simulink model "GPI1"  (Simulink 7.0)
settings: Solver=ode45  StartTime=0.0  StopTime=1000.0  RelTol=1e-3
values from neighbouring files (symbols this model uses):
  A_gpegpi = 1    [data_GPE.m]    (also in data_GPI.m)
  A_gpi = 2    [data_GPI.m]
  A_stngpi = 1    [data_GPI.m]    (also in data_STN.m)
  B_gpegpi = .1    (= 0.1)    [data_GPE.m]    (also in data_GPI.m)
  B_gpi = .08    (= 0.08)    [data_GPI.m]
  B_stngpi = .05    (= 0.05)    [data_GPI.m]    (also in data_STN.m)
  c_gpi = 1    [data_GPI.m]
  cagi0 = i_v_16(289:304)    [launch_sysGPI_mod.m]
  egpegpi = -100    [data_synapses.m]
  ek_gpi = -80.0    (= -80)    [data_GPI.m]
  el_gpi = -55.0    (= -55)    [data_GPI.m]
  epsil_gpi = 1*10^-4    (= 0.0001)    [data_GPI.m]
  estngpi = 0    [data_synapses.m]
  gahp_gpi = 30.0    (= 30)    [data_GPI.m]
  gca_gpi = 0.15    [data_GPI.m]
  ggpegpi = ggpegpi_vec(i)    [CN_launch_CN_analyze_TAL2.m]    (also in data_synapses.m = 1; launch_sysGPI_mod.m = 0.3)
  gk_gpi = 30.0    (= 30)    [data_GPI.m]
  gl_gpi = .1    (= 0.1)    [data_GPI.m]
  gna_gpi = 120    [data_GPI.m]
  gstngpi = .3    (= 0.3)    [data_synapses.m]
  gt_gpi = .5    (= 0.5)    [data_GPI.m]
  hgi0 = i_v_16(241:256)    [launch_sysGPI_mod.m]
  k1_gpi = 30.0    (= 30)    [data_GPI.m]
  kca_gpi = 15    [data_GPI.m]
  ngi0 = i_v_16(257:272)    [launch_sysGPI_mod.m]
  phih_gpi = 0.05    [data_GPI.m]
  phin_gpi = 0.1    [data_GPI.m]
  phir_gpi = 1    [data_GPI.m]
  rgi0 = i_v_16(273:288)    [launch_sysGPI_mod.m]
  sgi0 = i_v_16(305:320)    [launch_sysGPI_mod.m]
  sig0 = i_v_16(209:224)    [launch_sysGPI_mod.m]
  sigmaa_gpi = 2    [data_GPI.m]
  sigmagh_gpe = 2.0    (= 2)    [data_GPE.m]
  sigmagh_gpi = 2.0    (= 2)    [data_GPI.m]
  sigmagh_stn = 8.0    (= 8)    [data_STN.m]
  sigmah_gpi = -12    [data_GPI.m]
  sigmam_gpi = 10.0    (= 10)    [data_GPI.m]
  sigman_gpi = 14.0    (= 14)    [data_GPI.m]
  sigmar_gpi = -2.0    (= -2)    [data_GPI.m]
  sigmas_gpi = 2    [data_GPI.m]
  sigmatauh_gpi = -12    [data_GPI.m]
  sigmataun_gpi = -12.0    (= -12)    [data_GPI.m]
  sis0 = i_v_16(97:112)    [launch_sysGPI_mod.m]
  tauh0_gpi = .05    (= 0.05)    [data_GPI.m]
  tauh1_gpi = .27    (= 0.27)    [data_GPI.m]
  taun0_gpi = .05    (= 0.05)    [data_GPI.m]
  taun1_gpi = .27    (= 0.27)    [data_GPI.m]
  taur_gpi = 30.0    (= 30)    [data_GPI.m]
  theta_gpe = 20    [data_GPE.m]    (also in data_GPI.m)
  theta_gpi = 20    [data_GPI.m]
  theta_stn = 30    [data_GPI.m]    (also in data_STN.m)
  thetaa_gpi = -57.0    (= -57)    [data_GPI.m]
  thetagh_gpe = -57.0    (= -57)    [data_GPE.m]
  thetagh_gpi = -57.0    (= -57)    [data_GPI.m]
  thetagh_stn = -39.0    (= -39)    [data_STN.m]
  thetah_gpi = -58.0    (= -58)    [data_GPI.m]
  thetam_gpi = -37.0    (= -37)    [data_GPI.m]
  thetan_gpi = -50.0    (= -50)    [data_GPI.m]
  thetar_gpi = -70.0    (= -70)    [data_GPI.m]
  thetas_gpi = -35.0    (= -35)    [data_GPI.m]
  thetatauh_gpi = -40.0    (= -40)    [data_GPI.m]
  thetataun_gpi = -40.0    (= -40)    [data_GPI.m]
  vgi0 = i_v_16(225:240)    [launch_sysGPI_mod.m]
(part 6 of 6)

== system GPI1/gpicomp3/gpi_cell/ina/ina_gpi ==
  In1 : Inport  OutDataType=sfix(16)  OutScaling=2^0
  In2 : Inport  Port=2  OutDataType=sfix(16)  OutScaling=2^0
  In3 : Inport  Port=3  OutDataType=sfix(16)  OutScaling=2^0
  Fcn1 : Fcn  Expr=u^3*gna_gpi
  Fcn2 : Fcn  Expr=u-ena_gpi
  Product : Product  Inputs=3  OutDataType=sfix(16)  OutScaling=2^0  SaturateOnIntegerOverflow=on  InputSameDT=on
  Out1 : Outport  OutDataType=sfix(16)  OutScaling=2^0
  wires:
  Fcn1/1 -> Product/2
  Fcn2/1 -> Product/1
  In1/1 -> Fcn2/1
  Product/1 -> Out1/1
  In3/1 -> Product/3
  In2/1 -> Fcn1/1

== system GPI1/gpicomp3/gpi_cell/it/it_gpi ==
  In1 : Inport  OutDataType=sfix(16)  OutScaling=2^0
  In2 : Inport  Port=2  OutDataType=sfix(16)  OutScaling=2^0
  In3 : Inport  Port=3  OutDataType=sfix(16)  OutScaling=2^0
  Fcn1 : Fcn  Expr=u^2*gt_gpi
  Fcn2 : Fcn  Expr=u-eca_gpi
  Fcn3 : Fcn  Expr=u^3
  Product : Product  Inputs=3  OutDataType=sfix(16)  OutScaling=2^0  SaturateOnIntegerOverflow=on  InputSameDT=on
  Out1 : Outport  OutDataType=sfix(16)  OutScaling=2^0
  wires:
  Fcn1/1 -> Product/2
  Fcn2/1 -> Product/1
  In1/1 -> Fcn2/1
  Product/1 -> Out1/1
  In2/1 -> Fcn1/1
  In3/1 -> Fcn3/1
  Fcn3/1 -> Product/3

== system GPI1/gpicomp3/gpi_cell/it/r_gpi ==
  In1 : Inport  OutDataType=sfix(16)  OutScaling=2^0
  In2 : Inport  Port=2  OutDataType=sfix(16)  OutScaling=2^0
  1/tau_r : Fcn  Expr=1/taur_gpi
  Gain : Gain  Gain=phir_gpi  ParameterDataType=sfix(16)  ParameterScaling=2^0  OutDataType=sfix(16)  OutScaling=2^0  SaturateOnIntegerOverflow=on
  Integrator1 : Integrator  InitialConditionSource=external
  Product : Product  OutDataType=sfix(16)  OutScaling=2^0  SaturateOnIntegerOverflow=on  InputSameDT=on
  Sum1 : Sum  Inputs=|+-  OutDataType=sfix(16)  OutScaling=2^0  SaturateOnIntegerOverflow=on  InputSameDT=on
  rinf : Fcn  Expr=1/(1 + exp(-(u-thetar_gpi)/sigmar_gpi))
  Out1 : Outport  OutDataType=sfix(16)  OutScaling=2^0
  wires:
  In1/1 -> 1/tau_r/1, rinf/1
  1/tau_r/1 -> Product/1
  Integrator1/1 -> Sum1/2, Out1/1
  rinf/1 -> Sum1/1
  Sum1/1 -> Product/2
  Product/1 -> Gain/1
  Gain/1 -> Integrator1/1
  In2/1 -> Integrator1/2

== system GPI1/gpicomp4/gpi_cell/iahp/Subsystem ==
  In1 : Inport  OutDataType=sfix(16)  OutScaling=2^0
  In2 : Inport  Port=2  OutDataType=sfix(16)  OutScaling=2^0
  In3 : Inport  Port=3  OutDataType=sfix(16)  OutScaling=2^0
  Gain1 : Gain  Gain=epsil_gpi  ParameterDataType=sfix(16)  ParameterScaling=2^0  OutDataType=sfix(16)  OutScaling=2^0  SaturateOnIntegerOverflow=on
  Gain2 : Gain  Orientation=left  Gain=kca_gpi  ParameterDataType=sfix(16)  ParameterScaling=2^0  OutDataType=sfix(16)  OutScaling=2^0  SaturateOnIntegerOverflow=on
  Integrator1 : Integrator  InitialConditionSource=external  InitialCondition=0.03
  Sum1 : Sum  Inputs=---  OutDataType=sfix(16)  OutScaling=2^0  SaturateOnIntegerOverflow=on  InputSameDT=on
  Out1 : Outport  OutDataType=sfix(16)  OutScaling=2^0
  wires:
  Sum1/1 -> Gain1/1
  Gain1/1 -> Integrator1/1
  Gain2/1 -> Sum1/3
  Integrator1/1 -> Out1/1, Gain2/1
  In1/1 -> Sum1/1
  In2/1 -> Sum1/2
  In3/1 -> Integrator1/2

== system GPI1/gpicomp4/gpi_cell/ica/ica_gpe ==
  In1 : Inport  OutDataType=sfix(16)  OutScaling=2^0
  In2 : Inport  Port=2  OutDataType=sfix(16)  OutScaling=2^0
  Fcn1 : Fcn  Expr=u^2*gca_gpi
  Fcn2 : Fcn  Expr=u-eca_gpi
  Product : Product  OutDataType=sfix(16)  OutScaling=2^0  SaturateOnIntegerOverflow=on  InputSameDT=on
  Out1 : Outport  OutDataType=sfix(16)  OutScaling=2^0
  wires:
  Fcn1/1 -> Product/2
  Fcn2/1 -> Product/1
  In1/1 -> Fcn2/1
  Product/1 -> Out1/1
  In2/1 -> Fcn1/1

== system GPI1/gpicomp4/gpi_cell/ik/ik_gpi ==
  In1 : Inport  OutDataType=sfix(16)  OutScaling=2^0
  In2 : Inport  Port=2  OutDataType=sfix(16)  OutScaling=2^0
  Fcn1 : Fcn  Expr=u^4*gk_gpi
  Fcn2 : Fcn  Expr=u-ek_gpi
  Product : Product  OutDataType=sfix(16)  OutScaling=2^0  SaturateOnIntegerOverflow=on  InputSameDT=on
  Out1 : Outport  OutDataType=sfix(16)  OutScaling=2^0
  wires:
  Fcn1/1 -> Product/2
  Fcn2/1 -> Product/1
  In1/1 -> Fcn2/1
  Product/1 -> Out1/1
  In2/1 -> Fcn1/1

== system GPI1/gpicomp4/gpi_cell/ik/n_gpi ==
  In1 : Inport  OutDataType=sfix(16)  OutScaling=2^0
  In2 : Inport  Port=2  OutDataType=sfix(16)  OutScaling=2^0
  1/tau_n : Fcn  Expr=1/(taun0_gpi+ taun1_gpi/(1+exp(-(u-thetataun_gpi)/sigmataun_gpi)))
  Gain : Gain  Gain=phin_gpi  ParameterDataType=sfix(16)  ParameterScaling=2^0  OutDataType=sfix(16)  OutScaling=2^0  SaturateOnIntegerOverflow=on
  Integrator1 : Integrator  InitialConditionSource=external
  Product : Product  OutDataType=sfix(16)  OutScaling=2^0  SaturateOnIntegerOverflow=on  InputSameDT=on
  Sum1 : Sum  Inputs=|+-  OutDataType=sfix(16)  OutScaling=2^0  SaturateOnIntegerOverflow=on  InputSameDT=on
  ninf : Fcn  Expr=1/(1 + exp(-(u-thetan_gpi)/sigman_gpi))
  Out1 : Outport  OutDataType=sfix(16)  OutScaling=2^0
  wires:
  In1/1 -> 1/tau_n/1, ninf/1
  1/tau_n/1 -> Product/1
  Integrator1/1 -> Sum1/2, Out1/1
  ninf/1 -> Sum1/1
  Sum1/1 -> Product/2
  Product/1 -> Gain/1
  Gain/1 -> Integrator1/1
  In2/1 -> Integrator1/2

== system GPI1/gpicomp4/gpi_cell/ina/h_gpi ==
  In1 : Inport  OutDataType=sfix(16)  OutScaling=2^0
  In2 : Inport  Port=2  OutDataType=sfix(16)  OutScaling=2^0
  1/tau_h : Fcn  Expr=1/(tauh0_gpi + tauh1_gpi/(1+exp(-(u-thetatauh_gpi)/sigmatauh_gpi)))
  Gain : Gain  Gain=phih_gpi  ParameterDataType=sfix(16)  ParameterScaling=2^0  OutDataType=sfix(16)  OutScaling=2^0  SaturateOnIntegerOverflow=on
  Integrator1 : Integrator  InitialConditionSource=external
  Product : Product  OutDataType=sfix(16)  OutScaling=2^0  SaturateOnIntegerOverflow=on  InputSameDT=on
  Sum1 : Sum  Inputs=|+-  OutDataType=sfix(16)  OutScaling=2^0  SaturateOnIntegerOverflow=on  InputSameDT=on
  hinf : Fcn  Expr=1/(1 + exp(-(u-thetah_gpi)/sigmah_gpi))
  Out1 : Outport  OutDataType=sfix(16)  OutScaling=2^0
  wires:
  In1/1 -> 1/tau_h/1, hinf/1
  1/tau_h/1 -> Product/1
  Integrator1/1 -> Sum1/2, Out1/1
  hinf/1 -> Sum1/1
  Sum1/1 -> Product/2
  Product/1 -> Gain/1
  Gain/1 -> Integrator1/1
  In2/1 -> Integrator1/2

== system GPI1/gpicomp4/gpi_cell/ina/ina_gpi ==
  In1 : Inport  OutDataType=sfix(16)  OutScaling=2^0
  In2 : Inport  Port=2  OutDataType=sfix(16)  OutScaling=2^0
  In3 : Inport  Port=3  OutDataType=sfix(16)  OutScaling=2^0
  Fcn1 : Fcn  Expr=u^3*gna_gpi
  Fcn2 : Fcn  Expr=u-ena_gpi
  Product : Product  Inputs=3  OutDataType=sfix(16)  OutScaling=2^0  SaturateOnIntegerOverflow=on  InputSameDT=on
  Out1 : Outport  OutDataType=sfix(16)  OutScaling=2^0
  wires:
  Fcn1/1 -> Product/2
  Fcn2/1 -> Product/1
  In1/1 -> Fcn2/1
  Product/1 -> Out1/1
  In3/1 -> Product/3
  In2/1 -> Fcn1/1

== system GPI1/gpicomp4/gpi_cell/it/it_gpi ==
  In1 : Inport  OutDataType=sfix(16)  OutScaling=2^0
  In2 : Inport  Port=2  OutDataType=sfix(16)  OutScaling=2^0
  In3 : Inport  Port=3  OutDataType=sfix(16)  OutScaling=2^0
  Fcn1 : Fcn  Expr=u^2*gt_gpi
  Fcn2 : Fcn  Expr=u-eca_gpi
  Fcn3 : Fcn  Expr=u^3
  Product : Product  Inputs=3  OutDataType=sfix(16)  OutScaling=2^0  SaturateOnIntegerOverflow=on  InputSameDT=on
  Out1 : Outport  OutDataType=sfix(16)  OutScaling=2^0
  wires:
  Fcn1/1 -> Product/2
  Fcn2/1 -> Product/1
  In1/1 -> Fcn2/1
  Product/1 -> Out1/1
  In2/1 -> Fcn1/1
  In3/1 -> Fcn3/1
  Fcn3/1 -> Product/3

== system GPI1/gpicomp4/gpi_cell/it/r_gpi ==
  In1 : Inport  OutDataType=sfix(16)  OutScaling=2^0
  In2 : Inport  Port=2  OutDataType=sfix(16)  OutScaling=2^0
  1/tau_r : Fcn  Expr=1/taur_gpi
  Gain : Gain  Gain=phir_gpi  ParameterDataType=sfix(16)  ParameterScaling=2^0  OutDataType=sfix(16)  OutScaling=2^0  SaturateOnIntegerOverflow=on
  Integrator1 : Integrator  InitialConditionSource=external
  Product : Product  OutDataType=sfix(16)  OutScaling=2^0  SaturateOnIntegerOverflow=on  InputSameDT=on
  Sum1 : Sum  Inputs=|+-  OutDataType=sfix(16)  OutScaling=2^0  SaturateOnIntegerOverflow=on  InputSameDT=on
  rinf : Fcn  Expr=1/(1 + exp(-(u-thetar_gpi)/sigmar_gpi))
  Out1 : Outport  OutDataType=sfix(16)  OutScaling=2^0
  wires:
  In1/1 -> 1/tau_r/1, rinf/1
  1/tau_r/1 -> Product/1
  Integrator1/1 -> Sum1/2, Out1/1
  rinf/1 -> Sum1/1
  Sum1/1 -> Product/2
  Product/1 -> Gain/1
  Gain/1 -> Integrator1/1
  In2/1 -> Integrator1/2

== system GPI1/gpicomp5/gpi_cell/iahp/Subsystem ==
  In1 : Inport  OutDataType=sfix(16)  OutScaling=2^0
  In2 : Inport  Port=2  OutDataType=sfix(16)  OutScaling=2^0
  In3 : Inport  Port=3  OutDataType=sfix(16)  OutScaling=2^0
  Gain1 : Gain  Gain=epsil_gpi  ParameterDataType=sfix(16)  ParameterScaling=2^0  OutDataType=sfix(16)  OutScaling=2^0  SaturateOnIntegerOverflow=on
  Gain2 : Gain  Orientation=left  Gain=kca_gpi  ParameterDataType=sfix(16)  ParameterScaling=2^0  OutDataType=sfix(16)  OutScaling=2^0  SaturateOnIntegerOverflow=on
  Integrator1 : Integrator  InitialConditionSource=external  InitialCondition=0.03
  Sum1 : Sum  Inputs=---  OutDataType=sfix(16)  OutScaling=2^0  SaturateOnIntegerOverflow=on  InputSameDT=on
  Out1 : Outport  OutDataType=sfix(16)  OutScaling=2^0
  wires:
  Sum1/1 -> Gain1/1
  Gain1/1 -> Integrator1/1
  Gain2/1 -> Sum1/3
  Integrator1/1 -> Out1/1, Gain2/1
  In1/1 -> Sum1/1
  In2/1 -> Sum1/2
  In3/1 -> Integrator1/2

== system GPI1/gpicomp5/gpi_cell/ica/ica_gpe ==
  In1 : Inport  OutDataType=sfix(16)  OutScaling=2^0
  In2 : Inport  Port=2  OutDataType=sfix(16)  OutScaling=2^0
  Fcn1 : Fcn  Expr=u^2*gca_gpi
  Fcn2 : Fcn  Expr=u-eca_gpi
  Product : Product  OutDataType=sfix(16)  OutScaling=2^0  SaturateOnIntegerOverflow=on  InputSameDT=on
  Out1 : Outport  OutDataType=sfix(16)  OutScaling=2^0
  wires:
  Fcn1/1 -> Product/2
  Fcn2/1 -> Product/1
  In1/1 -> Fcn2/1
  Product/1 -> Out1/1
  In2/1 -> Fcn1/1

== system GPI1/gpicomp5/gpi_cell/ik/ik_gpi ==
  In1 : Inport  OutDataType=sfix(16)  OutScaling=2^0
  In2 : Inport  Port=2  OutDataType=sfix(16)  OutScaling=2^0
  Fcn1 : Fcn  Expr=u^4*gk_gpi
  Fcn2 : Fcn  Expr=u-ek_gpi
  Product : Product  OutDataType=sfix(16)  OutScaling=2^0  SaturateOnIntegerOverflow=on  InputSameDT=on
  Out1 : Outport  OutDataType=sfix(16)  OutScaling=2^0
  wires:
  Fcn1/1 -> Product/2
  Fcn2/1 -> Product/1
  In1/1 -> Fcn2/1
  Product/1 -> Out1/1
  In2/1 -> Fcn1/1

== system GPI1/gpicomp5/gpi_cell/ik/n_gpi ==
  In1 : Inport  OutDataType=sfix(16)  OutScaling=2^0
  In2 : Inport  Port=2  OutDataType=sfix(16)  OutScaling=2^0
  1/tau_n : Fcn  Expr=1/(taun0_gpi+ taun1_gpi/(1+exp(-(u-thetataun_gpi)/sigmataun_gpi)))
  Gain : Gain  Gain=phin_gpi  ParameterDataType=sfix(16)  ParameterScaling=2^0  OutDataType=sfix(16)  OutScaling=2^0  SaturateOnIntegerOverflow=on
  Integrator1 : Integrator  InitialConditionSource=external
  Product : Product  OutDataType=sfix(16)  OutScaling=2^0  SaturateOnIntegerOverflow=on  InputSameDT=on
  Sum1 : Sum  Inputs=|+-  OutDataType=sfix(16)  OutScaling=2^0  SaturateOnIntegerOverflow=on  InputSameDT=on
  ninf : Fcn  Expr=1/(1 + exp(-(u-thetan_gpi)/sigman_gpi))
  Out1 : Outport  OutDataType=sfix(16)  OutScaling=2^0
  wires:
  In1/1 -> 1/tau_n/1, ninf/1
  1/tau_n/1 -> Product/1
  Integrator1/1 -> Sum1/2, Out1/1
  ninf/1 -> Sum1/1
  Sum1/1 -> Product/2
  Product/1 -> Gain/1
  Gain/1 -> Integrator1/1
  In2/1 -> Integrator1/2

== system GPI1/gpicomp5/gpi_cell/ina/h_gpi ==
  In1 : Inport  OutDataType=sfix(16)  OutScaling=2^0
  In2 : Inport  Port=2  OutDataType=sfix(16)  OutScaling=2^0
  1/tau_h : Fcn  Expr=1/(tauh0_gpi + tauh1_gpi/(1+exp(-(u-thetatauh_gpi)/sigmatauh_gpi)))
  Gain : Gain  Gain=phih_gpi  ParameterDataType=sfix(16)  ParameterScaling=2^0  OutDataType=sfix(16)  OutScaling=2^0  SaturateOnIntegerOverflow=on
  Integrator1 : Integrator  InitialConditionSource=external
  Product : Product  OutDataType=sfix(16)  OutScaling=2^0  SaturateOnIntegerOverflow=on  InputSameDT=on
  Sum1 : Sum  Inputs=|+-  OutDataType=sfix(16)  OutScaling=2^0  SaturateOnIntegerOverflow=on  InputSameDT=on
  hinf : Fcn  Expr=1/(1 + exp(-(u-thetah_gpi)/sigmah_gpi))
  Out1 : Outport  OutDataType=sfix(16)  OutScaling=2^0
  wires:
  In1/1 -> 1/tau_h/1, hinf/1
  1/tau_h/1 -> Product/1
  Integrator1/1 -> Sum1/2, Out1/1
  hinf/1 -> Sum1/1
  Sum1/1 -> Product/2
  Product/1 -> Gain/1
  Gain/1 -> Integrator1/1
  In2/1 -> Integrator1/2

== system GPI1/gpicomp5/gpi_cell/ina/ina_gpi ==
  In1 : Inport  OutDataType=sfix(16)  OutScaling=2^0
  In2 : Inport  Port=2  OutDataType=sfix(16)  OutScaling=2^0
  In3 : Inport  Port=3  OutDataType=sfix(16)  OutScaling=2^0
  Fcn1 : Fcn  Expr=u^3*gna_gpi
  Fcn2 : Fcn  Expr=u-ena_gpi
  Product : Product  Inputs=3  OutDataType=sfix(16)  OutScaling=2^0  SaturateOnIntegerOverflow=on  InputSameDT=on
  Out1 : Outport  OutDataType=sfix(16)  OutScaling=2^0
  wires:
  Fcn1/1 -> Product/2
  Fcn2/1 -> Product/1
  In1/1 -> Fcn2/1
  Product/1 -> Out1/1
  In3/1 -> Product/3
  In2/1 -> Fcn1/1

== system GPI1/gpicomp5/gpi_cell/it/it_gpi ==
  In1 : Inport  OutDataType=sfix(16)  OutScaling=2^0
  In2 : Inport  Port=2  OutDataType=sfix(16)  OutScaling=2^0
  In3 : Inport  Port=3  OutDataType=sfix(16)  OutScaling=2^0
  Fcn1 : Fcn  Expr=u^2*gt_gpi
  Fcn2 : Fcn  Expr=u-eca_gpi
  Fcn3 : Fcn  Expr=u^3
  Product : Product  Inputs=3  OutDataType=sfix(16)  OutScaling=2^0  SaturateOnIntegerOverflow=on  InputSameDT=on
  Out1 : Outport  OutDataType=sfix(16)  OutScaling=2^0
  wires:
  Fcn1/1 -> Product/2
  Fcn2/1 -> Product/1
  In1/1 -> Fcn2/1
  Product/1 -> Out1/1
  In2/1 -> Fcn1/1
  In3/1 -> Fcn3/1
  Fcn3/1 -> Product/3

== system GPI1/gpicomp5/gpi_cell/it/r_gpi ==
  In1 : Inport  OutDataType=sfix(16)  OutScaling=2^0
  In2 : Inport  Port=2  OutDataType=sfix(16)  OutScaling=2^0
  1/tau_r : Fcn  Expr=1/taur_gpi
  Gain : Gain  Gain=phir_gpi  ParameterDataType=sfix(16)  ParameterScaling=2^0  OutDataType=sfix(16)  OutScaling=2^0  SaturateOnIntegerOverflow=on
  Integrator1 : Integrator  InitialConditionSource=external
  Product : Product  OutDataType=sfix(16)  OutScaling=2^0  SaturateOnIntegerOverflow=on  InputSameDT=on
  Sum1 : Sum  Inputs=|+-  OutDataType=sfix(16)  OutScaling=2^0  SaturateOnIntegerOverflow=on  InputSameDT=on
  rinf : Fcn  Expr=1/(1 + exp(-(u-thetar_gpi)/sigmar_gpi))
  Out1 : Outport  OutDataType=sfix(16)  OutScaling=2^0
  wires:
  In1/1 -> 1/tau_r/1, rinf/1
  1/tau_r/1 -> Product/1
  Integrator1/1 -> Sum1/2, Out1/1
  rinf/1 -> Sum1/1
  Sum1/1 -> Product/2
  Product/1 -> Gain/1
  Gain/1 -> Integrator1/1
  In2/1 -> Integrator1/2

== system GPI1/gpicomp6/gpi_cell/iahp/Subsystem ==
  In1 : Inport  OutDataType=sfix(16)  OutScaling=2^0
  In2 : Inport  Port=2  OutDataType=sfix(16)  OutScaling=2^0
  In3 : Inport  Port=3  OutDataType=sfix(16)  OutScaling=2^0
  Gain1 : Gain  Gain=epsil_gpi  ParameterDataType=sfix(16)  ParameterScaling=2^0  OutDataType=sfix(16)  OutScaling=2^0  SaturateOnIntegerOverflow=on
  Gain2 : Gain  Orientation=left  Gain=kca_gpi  ParameterDataType=sfix(16)  ParameterScaling=2^0  OutDataType=sfix(16)  OutScaling=2^0  SaturateOnIntegerOverflow=on
  Integrator1 : Integrator  InitialConditionSource=external  InitialCondition=0.03
  Sum1 : Sum  Inputs=---  OutDataType=sfix(16)  OutScaling=2^0  SaturateOnIntegerOverflow=on  InputSameDT=on
  Out1 : Outport  OutDataType=sfix(16)  OutScaling=2^0
  wires:
  Sum1/1 -> Gain1/1
  Gain1/1 -> Integrator1/1
  Gain2/1 -> Sum1/3
  Integrator1/1 -> Out1/1, Gain2/1
  In1/1 -> Sum1/1
  In2/1 -> Sum1/2
  In3/1 -> Integrator1/2

== system GPI1/gpicomp6/gpi_cell/ica/ica_gpe ==
  In1 : Inport  OutDataType=sfix(16)  OutScaling=2^0
  In2 : Inport  Port=2  OutDataType=sfix(16)  OutScaling=2^0
  Fcn1 : Fcn  Expr=u^2*gca_gpi
  Fcn2 : Fcn  Expr=u-eca_gpi
  Product : Product  OutDataType=sfix(16)  OutScaling=2^0  SaturateOnIntegerOverflow=on  InputSameDT=on
  Out1 : Outport  OutDataType=sfix(16)  OutScaling=2^0
  wires:
  Fcn1/1 -> Product/2
  Fcn2/1 -> Product/1
  In1/1 -> Fcn2/1
  Product/1 -> Out1/1
  In2/1 -> Fcn1/1

== system GPI1/gpicomp6/gpi_cell/ik/ik_gpi ==
  In1 : Inport  OutDataType=sfix(16)  OutScaling=2^0
  In2 : Inport  Port=2  OutDataType=sfix(16)  OutScaling=2^0
  Fcn1 : Fcn  Expr=u^4*gk_gpi
  Fcn2 : Fcn  Expr=u-ek_gpi
  Product : Product  OutDataType=sfix(16)  OutScaling=2^0  SaturateOnIntegerOverflow=on  InputSameDT=on
  Out1 : Outport  OutDataType=sfix(16)  OutScaling=2^0
  wires:
  Fcn1/1 -> Product/2
  Fcn2/1 -> Product/1
  In1/1 -> Fcn2/1
  Product/1 -> Out1/1
  In2/1 -> Fcn1/1

== system GPI1/gpicomp6/gpi_cell/ik/n_gpi ==
  In1 : Inport  OutDataType=sfix(16)  OutScaling=2^0
  In2 : Inport  Port=2  OutDataType=sfix(16)  OutScaling=2^0
  1/tau_n : Fcn  Expr=1/(taun0_gpi+ taun1_gpi/(1+exp(-(u-thetataun_gpi)/sigmataun_gpi)))
  Gain : Gain  Gain=phin_gpi  ParameterDataType=sfix(16)  ParameterScaling=2^0  OutDataType=sfix(16)  OutScaling=2^0  SaturateOnIntegerOverflow=on
  Integrator1 : Integrator  InitialConditionSource=external
  Product : Product  OutDataType=sfix(16)  OutScaling=2^0  SaturateOnIntegerOverflow=on  InputSameDT=on
  Sum1 : Sum  Inputs=|+-  OutDataType=sfix(16)  OutScaling=2^0  SaturateOnIntegerOverflow=on  InputSameDT=on
  ninf : Fcn  Expr=1/(1 + exp(-(u-thetan_gpi)/sigman_gpi))
  Out1 : Outport  OutDataType=sfix(16)  OutScaling=2^0
  wires:
  In1/1 -> 1/tau_n/1, ninf/1
  1/tau_n/1 -> Product/1
  Integrator1/1 -> Sum1/2, Out1/1
  ninf/1 -> Sum1/1
  Sum1/1 -> Product/2
  Product/1 -> Gain/1
  Gain/1 -> Integrator1/1
  In2/1 -> Integrator1/2

== system GPI1/gpicomp6/gpi_cell/ina/h_gpi ==
  In1 : Inport  OutDataType=sfix(16)  OutScaling=2^0
  In2 : Inport  Port=2  OutDataType=sfix(16)  OutScaling=2^0
  1/tau_h : Fcn  Expr=1/(tauh0_gpi + tauh1_gpi/(1+exp(-(u-thetatauh_gpi)/sigmatauh_gpi)))
  Gain : Gain  Gain=phih_gpi  ParameterDataType=sfix(16)  ParameterScaling=2^0  OutDataType=sfix(16)  OutScaling=2^0  SaturateOnIntegerOverflow=on
  Integrator1 : Integrator  InitialConditionSource=external
  Product : Product  OutDataType=sfix(16)  OutScaling=2^0  SaturateOnIntegerOverflow=on  InputSameDT=on
  Sum1 : Sum  Inputs=|+-  OutDataType=sfix(16)  OutScaling=2^0  SaturateOnIntegerOverflow=on  InputSameDT=on
  hinf : Fcn  Expr=1/(1 + exp(-(u-thetah_gpi)/sigmah_gpi))
  Out1 : Outport  OutDataType=sfix(16)  OutScaling=2^0
  wires:
  In1/1 -> 1/tau_h/1, hinf/1
  1/tau_h/1 -> Product/1
  Integrator1/1 -> Sum1/2, Out1/1
  hinf/1 -> Sum1/1
  Sum1/1 -> Product/2
  Product/1 -> Gain/1
  Gain/1 -> Integrator1/1
  In2/1 -> Integrator1/2

== system GPI1/gpicomp6/gpi_cell/ina/ina_gpi ==
  In1 : Inport  OutDataType=sfix(16)  OutScaling=2^0
  In2 : Inport  Port=2  OutDataType=sfix(16)  OutScaling=2^0
  In3 : Inport  Port=3  OutDataType=sfix(16)  OutScaling=2^0
  Fcn1 : Fcn  Expr=u^3*gna_gpi
  Fcn2 : Fcn  Expr=u-ena_gpi
  Product : Product  Inputs=3  OutDataType=sfix(16)  OutScaling=2^0  SaturateOnIntegerOverflow=on  InputSameDT=on
  Out1 : Outport  OutDataType=sfix(16)  OutScaling=2^0
  wires:
  Fcn1/1 -> Product/2
  Fcn2/1 -> Product/1
  In1/1 -> Fcn2/1
  Product/1 -> Out1/1
  In3/1 -> Product/3
  In2/1 -> Fcn1/1

== system GPI1/gpicomp6/gpi_cell/it/it_gpi ==
  In1 : Inport  OutDataType=sfix(16)  OutScaling=2^0
  In2 : Inport  Port=2  OutDataType=sfix(16)  OutScaling=2^0
  In3 : Inport  Port=3  OutDataType=sfix(16)  OutScaling=2^0
  Fcn1 : Fcn  Expr=u^2*gt_gpi
  Fcn2 : Fcn  Expr=u-eca_gpi
  Fcn3 : Fcn  Expr=u^3
  Product : Product  Inputs=3  OutDataType=sfix(16)  OutScaling=2^0  SaturateOnIntegerOverflow=on  InputSameDT=on
  Out1 : Outport  OutDataType=sfix(16)  OutScaling=2^0
  wires:
  Fcn1/1 -> Product/2
  Fcn2/1 -> Product/1
  In1/1 -> Fcn2/1
  Product/1 -> Out1/1
  In2/1 -> Fcn1/1
  In3/1 -> Fcn3/1
  Fcn3/1 -> Product/3

== system GPI1/gpicomp6/gpi_cell/it/r_gpi ==
  In1 : Inport  OutDataType=sfix(16)  OutScaling=2^0
  In2 : Inport  Port=2  OutDataType=sfix(16)  OutScaling=2^0
  1/tau_r : Fcn  Expr=1/taur_gpi
  Gain : Gain  Gain=phir_gpi  ParameterDataType=sfix(16)  ParameterScaling=2^0  OutDataType=sfix(16)  OutScaling=2^0  SaturateOnIntegerOverflow=on
  Integrator1 : Integrator  InitialConditionSource=external
  Product : Product  OutDataType=sfix(16)  OutScaling=2^0  SaturateOnIntegerOverflow=on  InputSameDT=on
  Sum1 : Sum  Inputs=|+-  OutDataType=sfix(16)  OutScaling=2^0  SaturateOnIntegerOverflow=on  InputSameDT=on
  rinf : Fcn  Expr=1/(1 + exp(-(u-thetar_gpi)/sigmar_gpi))
  Out1 : Outport  OutDataType=sfix(16)  OutScaling=2^0
  wires:
  In1/1 -> 1/tau_r/1, rinf/1
  1/tau_r/1 -> Product/1
  Integrator1/1 -> Sum1/2, Out1/1
  rinf/1 -> Sum1/1
  Sum1/1 -> Product/2
  Product/1 -> Gain/1
  Gain/1 -> Integrator1/1
  In2/1 -> Integrator1/2

== system GPI1/gpicomp7/gpi_cell/iahp/Subsystem ==
  In1 : Inport  OutDataType=sfix(16)  OutScaling=2^0
  In2 : Inport  Port=2  OutDataType=sfix(16)  OutScaling=2^0
  In3 : Inport  Port=3  OutDataType=sfix(16)  OutScaling=2^0
  Gain1 : Gain  Gain=epsil_gpi  ParameterDataType=sfix(16)  ParameterScaling=2^0  OutDataType=sfix(16)  OutScaling=2^0  SaturateOnIntegerOverflow=on
  Gain2 : Gain  Orientation=left  Gain=kca_gpi  ParameterDataType=sfix(16)  ParameterScaling=2^0  OutDataType=sfix(16)  OutScaling=2^0  SaturateOnIntegerOverflow=on
  Integrator1 : Integrator  InitialConditionSource=external  InitialCondition=0.03
  Sum1 : Sum  Inputs=---  OutDataType=sfix(16)  OutScaling=2^0  SaturateOnIntegerOverflow=on  InputSameDT=on
  Out1 : Outport  OutDataType=sfix(16)  OutScaling=2^0
  wires:
  Sum1/1 -> Gain1/1
  Gain1/1 -> Integrator1/1
  Gain2/1 -> Sum1/3
  Integrator1/1 -> Out1/1, Gain2/1
  In1/1 -> Sum1/1
  In2/1 -> Sum1/2
  In3/1 -> Integrator1/2

== system GPI1/gpicomp7/gpi_cell/ica/ica_gpe ==
  In1 : Inport  OutDataType=sfix(16)  OutScaling=2^0
  In2 : Inport  Port=2  OutDataType=sfix(16)  OutScaling=2^0
  Fcn1 : Fcn  Expr=u^2*gca_gpi
  Fcn2 : Fcn  Expr=u-eca_gpi
  Product : Product  OutDataType=sfix(16)  OutScaling=2^0  SaturateOnIntegerOverflow=on  InputSameDT=on
  Out1 : Outport  OutDataType=sfix(16)  OutScaling=2^0
  wires:
  Fcn1/1 -> Product/2
  Fcn2/1 -> Product/1
  In1/1 -> Fcn2/1
  Product/1 -> Out1/1
  In2/1 -> Fcn1/1

== system GPI1/gpicomp7/gpi_cell/ik/ik_gpi ==
  In1 : Inport  OutDataType=sfix(16)  OutScaling=2^0
  In2 : Inport  Port=2  OutDataType=sfix(16)  OutScaling=2^0
  Fcn1 : Fcn  Expr=u^4*gk_gpi
  Fcn2 : Fcn  Expr=u-ek_gpi
  Product : Product  OutDataType=sfix(16)  OutScaling=2^0  SaturateOnIntegerOverflow=on  InputSameDT=on
  Out1 : Outport  OutDataType=sfix(16)  OutScaling=2^0
  wires:
  Fcn1/1 -> Product/2
  Fcn2/1 -> Product/1
  In1/1 -> Fcn2/1
  Product/1 -> Out1/1
  In2/1 -> Fcn1/1

== system GPI1/gpicomp7/gpi_cell/ik/n_gpi ==
  In1 : Inport  OutDataType=sfix(16)  OutScaling=2^0
  In2 : Inport  Port=2  OutDataType=sfix(16)  OutScaling=2^0
  1/tau_n : Fcn  Expr=1/(taun0_gpi+ taun1_gpi/(1+exp(-(u-thetataun_gpi)/sigmataun_gpi)))
  Gain : Gain  Gain=phin_gpi  ParameterDataType=sfix(16)  ParameterScaling=2^0  OutDataType=sfix(16)  OutScaling=2^0  SaturateOnIntegerOverflow=on
  Integrator1 : Integrator  InitialConditionSource=external
  Product : Product  OutDataType=sfix(16)  OutScaling=2^0  SaturateOnIntegerOverflow=on  InputSameDT=on
  Sum1 : Sum  Inputs=|+-  OutDataType=sfix(16)  OutScaling=2^0  SaturateOnIntegerOverflow=on  InputSameDT=on
  ninf : Fcn  Expr=1/(1 + exp(-(u-thetan_gpi)/sigman_gpi))
  Out1 : Outport  OutDataType=sfix(16)  OutScaling=2^0
  wires:
  In1/1 -> 1/tau_n/1, ninf/1
  1/tau_n/1 -> Product/1
  Integrator1/1 -> Sum1/2, Out1/1
  ninf/1 -> Sum1/1
  Sum1/1 -> Product/2
  Product/1 -> Gain/1
  Gain/1 -> Integrator1/1
  In2/1 -> Integrator1/2

== system GPI1/gpicomp7/gpi_cell/ina/h_gpi ==
  In1 : Inport  OutDataType=sfix(16)  OutScaling=2^0
  In2 : Inport  Port=2  OutDataType=sfix(16)  OutScaling=2^0
  1/tau_h : Fcn  Expr=1/(tauh0_gpi + tauh1_gpi/(1+exp(-(u-thetatauh_gpi)/sigmatauh_gpi)))
  Gain : Gain  Gain=phih_gpi  ParameterDataType=sfix(16)  ParameterScaling=2^0  OutDataType=sfix(16)  OutScaling=2^0  SaturateOnIntegerOverflow=on
  Integrator1 : Integrator  InitialConditionSource=external
  Product : Product  OutDataType=sfix(16)  OutScaling=2^0  SaturateOnIntegerOverflow=on  InputSameDT=on
  Sum1 : Sum  Inputs=|+-  OutDataType=sfix(16)  OutScaling=2^0  SaturateOnIntegerOverflow=on  InputSameDT=on
  hinf : Fcn  Expr=1/(1 + exp(-(u-thetah_gpi)/sigmah_gpi))
  Out1 : Outport  OutDataType=sfix(16)  OutScaling=2^0
  wires:
  In1/1 -> 1/tau_h/1, hinf/1
  1/tau_h/1 -> Product/1
  Integrator1/1 -> Sum1/2, Out1/1
  hinf/1 -> Sum1/1
  Sum1/1 -> Product/2
  Product/1 -> Gain/1
  Gain/1 -> Integrator1/1
  In2/1 -> Integrator1/2

== system GPI1/gpicomp7/gpi_cell/ina/ina_gpi ==
  In1 : Inport  OutDataType=sfix(16)  OutScaling=2^0
  In2 : Inport  Port=2  OutDataType=sfix(16)  OutScaling=2^0
  In3 : Inport  Port=3  OutDataType=sfix(16)  OutScaling=2^0
  Fcn1 : Fcn  Expr=u^3*gna_gpi
  Fcn2 : Fcn  Expr=u-ena_gpi
  Product : Product  Inputs=3  OutDataType=sfix(16)  OutScaling=2^0  SaturateOnIntegerOverflow=on  InputSameDT=on
  Out1 : Outport  OutDataType=sfix(16)  OutScaling=2^0
  wires:
  Fcn1/1 -> Product/2
  Fcn2/1 -> Product/1
  In1/1 -> Fcn2/1
  Product/1 -> Out1/1
  In3/1 -> Product/3
  In2/1 -> Fcn1/1

== system GPI1/gpicomp7/gpi_cell/it/it_gpi ==
  In1 : Inport  OutDataType=sfix(16)  OutScaling=2^0
  In2 : Inport  Port=2  OutDataType=sfix(16)  OutScaling=2^0
  In3 : Inport  Port=3  OutDataType=sfix(16)  OutScaling=2^0
  Fcn1 : Fcn  Expr=u^2*gt_gpi
  Fcn2 : Fcn  Expr=u-eca_gpi
  Fcn3 : Fcn  Expr=u^3
  Product : Product  Inputs=3  OutDataType=sfix(16)  OutScaling=2^0  SaturateOnIntegerOverflow=on  InputSameDT=on
  Out1 : Outport  OutDataType=sfix(16)  OutScaling=2^0
  wires:
  Fcn1/1 -> Product/2
  Fcn2/1 -> Product/1
  In1/1 -> Fcn2/1
  Product/1 -> Out1/1
  In2/1 -> Fcn1/1
  In3/1 -> Fcn3/1
  Fcn3/1 -> Product/3

== system GPI1/gpicomp7/gpi_cell/it/r_gpi ==
  In1 : Inport  OutDataType=sfix(16)  OutScaling=2^0
  In2 : Inport  Port=2  OutDataType=sfix(16)  OutScaling=2^0
  1/tau_r : Fcn  Expr=1/taur_gpi
  Gain : Gain  Gain=phir_gpi  ParameterDataType=sfix(16)  ParameterScaling=2^0  OutDataType=sfix(16)  OutScaling=2^0  SaturateOnIntegerOverflow=on
  Integrator1 : Integrator  InitialConditionSource=external
  Product : Product  OutDataType=sfix(16)  OutScaling=2^0  SaturateOnIntegerOverflow=on  InputSameDT=on
  Sum1 : Sum  Inputs=|+-  OutDataType=sfix(16)  OutScaling=2^0  SaturateOnIntegerOverflow=on  InputSameDT=on
  rinf : Fcn  Expr=1/(1 + exp(-(u-thetar_gpi)/sigmar_gpi))
  Out1 : Outport  OutDataType=sfix(16)  OutScaling=2^0
  wires:
  In1/1 -> 1/tau_r/1, rinf/1
  1/tau_r/1 -> Product/1
  Integrator1/1 -> Sum1/2, Out1/1
  rinf/1 -> Sum1/1
  Sum1/1 -> Product/2
  Product/1 -> Gain/1
  Gain/1 -> Integrator1/1
  In2/1 -> Integrator1/2

== system GPI1/gpicomp8/gpi_cell/iahp/Subsystem ==
  In1 : Inport  OutDataType=sfix(16)  OutScaling=2^0
  In2 : Inport  Port=2  OutDataType=sfix(16)  OutScaling=2^0
  In3 : Inport  Port=3  OutDataType=sfix(16)  OutScaling=2^0
  Gain1 : Gain  Gain=epsil_gpi  ParameterDataType=sfix(16)  ParameterScaling=2^0  OutDataType=sfix(16)  OutScaling=2^0  SaturateOnIntegerOverflow=on
  Gain2 : Gain  Orientation=left  Gain=kca_gpi  ParameterDataType=sfix(16)  ParameterScaling=2^0  OutDataType=sfix(16)  OutScaling=2^0  SaturateOnIntegerOverflow=on
  Integrator1 : Integrator  InitialConditionSource=external  InitialCondition=0.03
  Sum1 : Sum  Inputs=---  OutDataType=sfix(16)  OutScaling=2^0  SaturateOnIntegerOverflow=on  InputSameDT=on
  Out1 : Outport  OutDataType=sfix(16)  OutScaling=2^0
  wires:
  Sum1/1 -> Gain1/1
  Gain1/1 -> Integrator1/1
  Gain2/1 -> Sum1/3
  Integrator1/1 -> Out1/1, Gain2/1
  In1/1 -> Sum1/1
  In2/1 -> Sum1/2
  In3/1 -> Integrator1/2

== system GPI1/gpicomp8/gpi_cell/ica/ica_gpe ==
  In1 : Inport  OutDataType=sfix(16)  OutScaling=2^0
  In2 : Inport  Port=2  OutDataType=sfix(16)  OutScaling=2^0
  Fcn1 : Fcn  Expr=u^2*gca_gpi
  Fcn2 : Fcn  Expr=u-eca_gpi
  Product : Product  OutDataType=sfix(16)  OutScaling=2^0  SaturateOnIntegerOverflow=on  InputSameDT=on
  Out1 : Outport  OutDataType=sfix(16)  OutScaling=2^0
  wires:
  Fcn1/1 -> Product/2
  Fcn2/1 -> Product/1
  In1/1 -> Fcn2/1
  Product/1 -> Out1/1
  In2/1 -> Fcn1/1

== system GPI1/gpicomp8/gpi_cell/ik/ik_gpi ==
  In1 : Inport  OutDataType=sfix(16)  OutScaling=2^0
  In2 : Inport  Port=2  OutDataType=sfix(16)  OutScaling=2^0
  Fcn1 : Fcn  Expr=u^4*gk_gpi
  Fcn2 : Fcn  Expr=u-ek_gpi
  Product : Product  OutDataType=sfix(16)  OutScaling=2^0  SaturateOnIntegerOverflow=on  InputSameDT=on
  Out1 : Outport  OutDataType=sfix(16)  OutScaling=2^0
  wires:
  Fcn1/1 -> Product/2
  Fcn2/1 -> Product/1
  In1/1 -> Fcn2/1
  Product/1 -> Out1/1
  In2/1 -> Fcn1/1

== system GPI1/gpicomp8/gpi_cell/ik/n_gpi ==
  In1 : Inport  OutDataType=sfix(16)  OutScaling=2^0
  In2 : Inport  Port=2  OutDataType=sfix(16)  OutScaling=2^0
  1/tau_n : Fcn  Expr=1/(taun0_gpi+ taun1_gpi/(1+exp(-(u-thetataun_gpi)/sigmataun_gpi)))
  Gain : Gain  Gain=phin_gpi  ParameterDataType=sfix(16)  ParameterScaling=2^0  OutDataType=sfix(16)  OutScaling=2^0  SaturateOnIntegerOverflow=on
  Integrator1 : Integrator  InitialConditionSource=external
  Product : Product  OutDataType=sfix(16)  OutScaling=2^0  SaturateOnIntegerOverflow=on  InputSameDT=on
  Sum1 : Sum  Inputs=|+-  OutDataType=sfix(16)  OutScaling=2^0  SaturateOnIntegerOverflow=on  InputSameDT=on
  ninf : Fcn  Expr=1/(1 + exp(-(u-thetan_gpi)/sigman_gpi))
  Out1 : Outport  OutDataType=sfix(16)  OutScaling=2^0
  wires:
  In1/1 -> 1/tau_n/1, ninf/1
  1/tau_n/1 -> Product/1
  Integrator1/1 -> Sum1/2, Out1/1
  ninf/1 -> Sum1/1
  Sum1/1 -> Product/2
  Product/1 -> Gain/1
  Gain/1 -> Integrator1/1
  In2/1 -> Integrator1/2

== system GPI1/gpicomp8/gpi_cell/ina/h_gpi ==
  In1 : Inport  OutDataType=sfix(16)  OutScaling=2^0
  In2 : Inport  Port=2  OutDataType=sfix(16)  OutScaling=2^0
  1/tau_h : Fcn  Expr=1/(tauh0_gpi + tauh1_gpi/(1+exp(-(u-thetatauh_gpi)/sigmatauh_gpi)))
  Gain : Gain  Gain=phih_gpi  ParameterDataType=sfix(16)  ParameterScaling=2^0  OutDataType=sfix(16)  OutScaling=2^0  SaturateOnIntegerOverflow=on
  Integrator1 : Integrator  InitialConditionSource=external
  Product : Product  OutDataType=sfix(16)  OutScaling=2^0  SaturateOnIntegerOverflow=on  InputSameDT=on
  Sum1 : Sum  Inputs=|+-  OutDataType=sfix(16)  OutScaling=2^0  SaturateOnIntegerOverflow=on  InputSameDT=on
  hinf : Fcn  Expr=1/(1 + exp(-(u-thetah_gpi)/sigmah_gpi))
  Out1 : Outport  OutDataType=sfix(16)  OutScaling=2^0
  wires:
  In1/1 -> 1/tau_h/1, hinf/1
  1/tau_h/1 -> Product/1
  Integrator1/1 -> Sum1/2, Out1/1
  hinf/1 -> Sum1/1
  Sum1/1 -> Product/2
  Product/1 -> Gain/1
  Gain/1 -> Integrator1/1
  In2/1 -> Integrator1/2

== system GPI1/gpicomp8/gpi_cell/ina/ina_gpi ==
  In1 : Inport  OutDataType=sfix(16)  OutScaling=2^0
  In2 : Inport  Port=2  OutDataType=sfix(16)  OutScaling=2^0
  In3 : Inport  Port=3  OutDataType=sfix(16)  OutScaling=2^0
  Fcn1 : Fcn  Expr=u^3*gna_gpi
  Fcn2 : Fcn  Expr=u-ena_gpi
  Product : Product  Inputs=3  OutDataType=sfix(16)  OutScaling=2^0  SaturateOnIntegerOverflow=on  InputSameDT=on
  Out1 : Outport  OutDataType=sfix(16)  OutScaling=2^0
  wires:
  Fcn1/1 -> Product/2
  Fcn2/1 -> Product/1
  In1/1 -> Fcn2/1
  Product/1 -> Out1/1
  In3/1 -> Product/3
  In2/1 -> Fcn1/1

== system GPI1/gpicomp8/gpi_cell/it/it_gpi ==
  In1 : Inport  OutDataType=sfix(16)  OutScaling=2^0
  In2 : Inport  Port=2  OutDataType=sfix(16)  OutScaling=2^0
  In3 : Inport  Port=3  OutDataType=sfix(16)  OutScaling=2^0
  Fcn1 : Fcn  Expr=u^2*gt_gpi
  Fcn2 : Fcn  Expr=u-eca_gpi
  Fcn3 : Fcn  Expr=u^3
  Product : Product  Inputs=3  OutDataType=sfix(16)  OutScaling=2^0  SaturateOnIntegerOverflow=on  InputSameDT=on
  Out1 : Outport  OutDataType=sfix(16)  OutScaling=2^0
  wires:
  Fcn1/1 -> Product/2
  Fcn2/1 -> Product/1
  In1/1 -> Fcn2/1
  Product/1 -> Out1/1
  In2/1 -> Fcn1/1
  In3/1 -> Fcn3/1
  Fcn3/1 -> Product/3

== system GPI1/gpicomp8/gpi_cell/it/r_gpi ==
  In1 : Inport  OutDataType=sfix(16)  OutScaling=2^0
  In2 : Inport  Port=2  OutDataType=sfix(16)  OutScaling=2^0
  1/tau_r : Fcn  Expr=1/taur_gpi
  Gain : Gain  Gain=phir_gpi  ParameterDataType=sfix(16)  ParameterScaling=2^0  OutDataType=sfix(16)  OutScaling=2^0  SaturateOnIntegerOverflow=on
  Integrator1 : Integrator  InitialConditionSource=external
  Product : Product  OutDataType=sfix(16)  OutScaling=2^0  SaturateOnIntegerOverflow=on  InputSameDT=on
  Sum1 : Sum  Inputs=|+-  OutDataType=sfix(16)  OutScaling=2^0  SaturateOnIntegerOverflow=on  InputSameDT=on
  rinf : Fcn  Expr=1/(1 + exp(-(u-thetar_gpi)/sigmar_gpi))
  Out1 : Outport  OutDataType=sfix(16)  OutScaling=2^0
  wires:
  In1/1 -> 1/tau_r/1, rinf/1
  1/tau_r/1 -> Product/1
  Integrator1/1 -> Sum1/2, Out1/1
  rinf/1 -> Sum1/1
  Sum1/1 -> Product/2
  Product/1 -> Gain/1
  Gain/1 -> Integrator1/1
  In2/1 -> Integrator1/2

== system GPI1/gpicomp9/gpi_cell/iahp/Subsystem ==
  In1 : Inport  OutDataType=sfix(16)  OutScaling=2^0
  In2 : Inport  Port=2  OutDataType=sfix(16)  OutScaling=2^0
  In3 : Inport  Port=3  OutDataType=sfix(16)  OutScaling=2^0
  Gain1 : Gain  Gain=epsil_gpi  ParameterDataType=sfix(16)  ParameterScaling=2^0  OutDataType=sfix(16)  OutScaling=2^0  SaturateOnIntegerOverflow=on
  Gain2 : Gain  Orientation=left  Gain=kca_gpi  ParameterDataType=sfix(16)  ParameterScaling=2^0  OutDataType=sfix(16)  OutScaling=2^0  SaturateOnIntegerOverflow=on
  Integrator1 : Integrator  InitialConditionSource=external  InitialCondition=0.03
  Sum1 : Sum  Inputs=---  OutDataType=sfix(16)  OutScaling=2^0  SaturateOnIntegerOverflow=on  InputSameDT=on
  Out1 : Outport  OutDataType=sfix(16)  OutScaling=2^0
  wires:
  Sum1/1 -> Gain1/1
  Gain1/1 -> Integrator1/1
  Gain2/1 -> Sum1/3
  Integrator1/1 -> Out1/1, Gain2/1
  In1/1 -> Sum1/1
  In2/1 -> Sum1/2
  In3/1 -> Integrator1/2

== system GPI1/gpicomp9/gpi_cell/ica/ica_gpe ==
  In1 : Inport  OutDataType=sfix(16)  OutScaling=2^0
  In2 : Inport  Port=2  OutDataType=sfix(16)  OutScaling=2^0
  Fcn1 : Fcn  Expr=u^2*gca_gpi
  Fcn2 : Fcn  Expr=u-eca_gpi
  Product : Product  OutDataType=sfix(16)  OutScaling=2^0  SaturateOnIntegerOverflow=on  InputSameDT=on
  Out1 : Outport  OutDataType=sfix(16)  OutScaling=2^0
  wires:
  Fcn1/1 -> Product/2
  Fcn2/1 -> Product/1
  In1/1 -> Fcn2/1
  Product/1 -> Out1/1
  In2/1 -> Fcn1/1

== system GPI1/gpicomp9/gpi_cell/ik/ik_gpi ==
  In1 : Inport  OutDataType=sfix(16)  OutScaling=2^0
  In2 : Inport  Port=2  OutDataType=sfix(16)  OutScaling=2^0
  Fcn1 : Fcn  Expr=u^4*gk_gpi
  Fcn2 : Fcn  Expr=u-ek_gpi
  Product : Product  OutDataType=sfix(16)  OutScaling=2^0  SaturateOnIntegerOverflow=on  InputSameDT=on
  Out1 : Outport  OutDataType=sfix(16)  OutScaling=2^0
  wires:
  Fcn1/1 -> Product/2
  Fcn2/1 -> Product/1
  In1/1 -> Fcn2/1
  Product/1 -> Out1/1
  In2/1 -> Fcn1/1

== system GPI1/gpicomp9/gpi_cell/ik/n_gpi ==
  In1 : Inport  OutDataType=sfix(16)  OutScaling=2^0
  In2 : Inport  Port=2  OutDataType=sfix(16)  OutScaling=2^0
  1/tau_n : Fcn  Expr=1/(taun0_gpi+ taun1_gpi/(1+exp(-(u-thetataun_gpi)/sigmataun_gpi)))
  Gain : Gain  Gain=phin_gpi  ParameterDataType=sfix(16)  ParameterScaling=2^0  OutDataType=sfix(16)  OutScaling=2^0  SaturateOnIntegerOverflow=on
  Integrator1 : Integrator  InitialConditionSource=external
  Product : Product  OutDataType=sfix(16)  OutScaling=2^0  SaturateOnIntegerOverflow=on  InputSameDT=on
  Sum1 : Sum  Inputs=|+-  OutDataType=sfix(16)  OutScaling=2^0  SaturateOnIntegerOverflow=on  InputSameDT=on
  ninf : Fcn  Expr=1/(1 + exp(-(u-thetan_gpi)/sigman_gpi))
  Out1 : Outport  OutDataType=sfix(16)  OutScaling=2^0
  wires:
  In1/1 -> 1/tau_n/1, ninf/1
  1/tau_n/1 -> Product/1
  Integrator1/1 -> Sum1/2, Out1/1
  ninf/1 -> Sum1/1
  Sum1/1 -> Product/2
  Product/1 -> Gain/1
  Gain/1 -> Integrator1/1
  In2/1 -> Integrator1/2

== system GPI1/gpicomp9/gpi_cell/ina/h_gpi ==
  In1 : Inport  OutDataType=sfix(16)  OutScaling=2^0
  In2 : Inport  Port=2  OutDataType=sfix(16)  OutScaling=2^0
  1/tau_h : Fcn  Expr=1/(tauh0_gpi + tauh1_gpi/(1+exp(-(u-thetatauh_gpi)/sigmatauh_gpi)))
  Gain : Gain  Gain=phih_gpi  ParameterDataType=sfix(16)  ParameterScaling=2^0  OutDataType=sfix(16)  OutScaling=2^0  SaturateOnIntegerOverflow=on
  Integrator1 : Integrator  InitialConditionSource=external
  Product : Product  OutDataType=sfix(16)  OutScaling=2^0  SaturateOnIntegerOverflow=on  InputSameDT=on
  Sum1 : Sum  Inputs=|+-  OutDataType=sfix(16)  OutScaling=2^0  SaturateOnIntegerOverflow=on  InputSameDT=on
  hinf : Fcn  Expr=1/(1 + exp(-(u-thetah_gpi)/sigmah_gpi))
  Out1 : Outport  OutDataType=sfix(16)  OutScaling=2^0
  wires:
  In1/1 -> 1/tau_h/1, hinf/1
  1/tau_h/1 -> Product/1
  Integrator1/1 -> Sum1/2, Out1/1
  hinf/1 -> Sum1/1
  Sum1/1 -> Product/2
  Product/1 -> Gain/1
  Gain/1 -> Integrator1/1
  In2/1 -> Integrator1/2

== system GPI1/gpicomp9/gpi_cell/ina/ina_gpi ==
  In1 : Inport  OutDataType=sfix(16)  OutScaling=2^0
  In2 : Inport  Port=2  OutDataType=sfix(16)  OutScaling=2^0
  In3 : Inport  Port=3  OutDataType=sfix(16)  OutScaling=2^0
  Fcn1 : Fcn  Expr=u^3*gna_gpi
  Fcn2 : Fcn  Expr=u-ena_gpi
  Product : Product  Inputs=3  OutDataType=sfix(16)  OutScaling=2^0  SaturateOnIntegerOverflow=on  InputSameDT=on
  Out1 : Outport  OutDataType=sfix(16)  OutScaling=2^0
  wires:
  Fcn1/1 -> Product/2
  Fcn2/1 -> Product/1
  In1/1 -> Fcn2/1
  Product/1 -> Out1/1
  In3/1 -> Product/3
  In2/1 -> Fcn1/1

== system GPI1/gpicomp9/gpi_cell/it/it_gpi ==
  In1 : Inport  OutDataType=sfix(16)  OutScaling=2^0
  In2 : Inport  Port=2  OutDataType=sfix(16)  OutScaling=2^0
  In3 : Inport  Port=3  OutDataType=sfix(16)  OutScaling=2^0
  Fcn1 : Fcn  Expr=u^2*gt_gpi
  Fcn2 : Fcn  Expr=u-eca_gpi
  Fcn3 : Fcn  Expr=u^3
  Product : Product  Inputs=3  OutDataType=sfix(16)  OutScaling=2^0  SaturateOnIntegerOverflow=on  InputSameDT=on
  Out1 : Outport  OutDataType=sfix(16)  OutScaling=2^0
  wires:
  Fcn1/1 -> Product/2
  Fcn2/1 -> Product/1
  In1/1 -> Fcn2/1
  Product/1 -> Out1/1
  In2/1 -> Fcn1/1
  In3/1 -> Fcn3/1
  Fcn3/1 -> Product/3

== system GPI1/gpicomp9/gpi_cell/it/r_gpi ==
  In1 : Inport  OutDataType=sfix(16)  OutScaling=2^0
  In2 : Inport  Port=2  OutDataType=sfix(16)  OutScaling=2^0
  1/tau_r : Fcn  Expr=1/taur_gpi
  Gain : Gain  Gain=phir_gpi  ParameterDataType=sfix(16)  ParameterScaling=2^0  OutDataType=sfix(16)  OutScaling=2^0  SaturateOnIntegerOverflow=on
  Integrator1 : Integrator  InitialConditionSource=external
  Product : Product  OutDataType=sfix(16)  OutScaling=2^0  SaturateOnIntegerOverflow=on  InputSameDT=on
  Sum1 : Sum  Inputs=|+-  OutDataType=sfix(16)  OutScaling=2^0  SaturateOnIntegerOverflow=on  InputSameDT=on
  rinf : Fcn  Expr=1/(1 + exp(-(u-thetar_gpi)/sigmar_gpi))
  Out1 : Outport  OutDataType=sfix(16)  OutScaling=2^0
  wires:
  In1/1 -> 1/tau_r/1, rinf/1
  1/tau_r/1 -> Product/1
  Integrator1/1 -> Sum1/2, Out1/1
  rinf/1 -> Sum1/1
  Sum1/1 -> Product/2
  Product/1 -> Gain/1
  Gain/1 -> Integrator1/1
  In2/1 -> Integrator1/2
